simulink model "AssembledTEST1"  (R2016b)
settings: Solver=VariableStepAuto  StartTime=0.0  StopTime=60  RelTol=1e-9
values from neighbouring files (symbols this model uses):
  DOWN_0 = -xtrim(12)    [Comparison_NonLin.m]    (also in InitialiseJ31.m = 1830.0192; Trim.m)
  EAST_0 = xtrim(11)    [Comparison_NonLin.m]    (also in InitialiseJ31.m = 0; Trim.m)
  FLAP = 0    [InitialiseJ31.m]
  INERTIA = [IXX,IXY,IXZ;IXY,IYY,IYZ;IXZ,IYZ,IZZ]    [InitialiseJ31.m]
  NORTH_0 = xtrim(10)    [Comparison_NonLin.m]    (also in InitialiseJ31.m = 0; Trim.m)
  P_0 = xtrim(4)    [Comparison_NonLin.m]    (also in InitialiseJ31.m = 0; Trim.m)
  PHI_0 = xtrim(7)    [Comparison_NonLin.m]    (also in Trim.m)
  PSI_0 = xtrim(9)    [Comparison_NonLin.m]    (also in Trim.m)
  Q_0 = xtrim(5)    [Comparison_NonLin.m]    (also in InitialiseJ31.m = 0; Trim.m)
  R2D = 180/pi    (= 57.2957795131)    [InitialiseJ31.m]
  R_0 = xtrim(6)    [Comparison_NonLin.m]    (also in InitialiseJ31.m = 0; Trim.m)
  THETA_0 = xtrim(8)    [Comparison_NonLin.m]    (also in Trim.m)
  U_0 = xtrim(1)    [Comparison_NonLin.m]    (also in Trim.m)
  V_0 = xtrim(2)    [Comparison_NonLin.m]    (also in Trim.m)
  W_0 = xtrim(3)    [Comparison_NonLin.m]    (also in Trim.m)
undefined symbols (not defined in the file or in its folder): ail_data, Ap, Aw, b, beta0_data, c0, c_i, cdrag_data, CG, clean_wing_data, crt, CT_data, D, D0q_10, D0q_20, D0q_35, DCDi_data, DCM0b, Deh_f_on_data, Deh_on_data, df, Dqhq_data, e0, e_data10, e_data20, e_data35, elaw_0, elaw_1, elaw_2, flaps_lift_data, flaps_moment_data, flaps_tail_data, flaps_wing_data, fmc_data, fmf_data, fmn_data, fus_data, gamma_t, h_data10, h_data20, h_data35, it, iw, Iwn2, J_W, K1_data, k1f_data, k_data, L_r0_10f, L_r0_20f, L_r0_35f, l_t, ld_data, Lt, Lt_dash, Lv_b, Lv_h, Lv_n, mac, mach_ffr ... (+39)
libraries: aerolibasang x3, aerolibatmos2 x1
(part 4 of 5)

== system AssembledTEST1/Subsystem/Powerplants and Slipstream/Subsystem2/Powerplant - port (forces and moments about spinner) (in body axes)/Get_Del_qhq ==
  ab : Inport
  In2 : Inport  Port=2
  eh : Inport  Port=3
  In3 : Inport  Port=4
  eu : Inport  Port=5
  ep : Inport  Port=6
  Abs : Abs
  Add : Sum  Inputs=+-+
  Add2 : Sum  Inputs=--+
  Constant1 : Constant  Value=Xp_dash
  Constant2 : Constant  Value=Lt_dash
  Constant3 : Constant  Value=Z_ht
  Constant4 : Constant  Value=D
  Constant5 : Constant  Value=2
  Constant6 : Constant  Value=Iwn2
  Divide : Product  Inputs=**/
  Embedded MATLAB Function : MATLAB Function  TreatAsAtomicUnit=on
  Embedded MATLAB Function1 : MATLAB Function  TreatAsAtomicUnit=on
  Fcn : Fcn  Expr=tan(u(1))
  Fcn1 : Fcn  Expr=tan(u(1))
  GetDehPower : Lookup2D  RowIndex=eh_off_ords  ColumnIndex=Tc2_ords  Table=Deh_on_data
  GetDehPower_flap : Lookup2D  RowIndex=eh_off_ords  ColumnIndex=Tc2_ords  Table=Deh_f_on_data
  GetDelqhq : Lookup2D  RowIndex=Zh_eff_ords  ColumnIndex=Tc3_ords  Table=Dqhq_data
  Product : Product  RndMeth=Zero
  Product1 : Product  RndMeth=Zero
  Saturation : Saturate  UpperLimit=10  LowerLimit=0  ZeroCross=off
  Saturation1 : Saturate  UpperLimit=2  LowerLimit=0  ZeroCross=off
  deg2rad : Gain  Gain=pi/180
  get_Zh_eff : Sum  Inputs=+-+
  rad2deg : Gain  Gain=180/pi
  Out1 : Outport
  Out2 : Outport  Port=2
  Out3 : Outport  Port=3
  wires:
  In3/1 -> GetDehPower_flap/2, GetDehPower/2, GetDelqhq/2, Embedded MATLAB Function1/3(TC)
  GetDehPower/1 -> Embedded MATLAB Function/2(Deh_power)
  GetDehPower_flap/1 -> Embedded MATLAB Function/3(Deh_power_flap)
  In2/1 -> Embedded MATLAB Function/1(Flap)
  rad2deg/1 -> GetDehPower/1, GetDehPower_flap/1
  eh/1 -> rad2deg/1, Add2/2
  eu/1 -> Add/1, Embedded MATLAB Function1/2(eu)
  ep/1 -> Add/2, Embedded MATLAB Function1/1(ep)
  ab/1 -> Add/3
  deg2rad/1 -> Add2/1, Out2/1
  Add/1 -> Fcn/1, Add2/3
  Constant1/1 -> Product/1
  Fcn/1 -> Product/2
  Add2/1 -> Fcn1/1
  Constant2/1 -> Product1/1
  Fcn1/1 -> Product1/2
  Product1/1 -> get_Zh_eff/1
  Constant3/1 -> get_Zh_eff/2
  Product/1 -> get_Zh_eff/3
  get_Zh_eff/1 -> Abs/1
  Embedded MATLAB Function/1(Del_eh_power) -> Saturation/1
  Saturation/1 -> deg2rad/1
  Abs/1 -> Divide/1
  Constant5/1 -> Divide/2
  Constant4/1 -> Divide/3
  Divide/1 -> GetDelqhq/1
  GetDelqhq/1 -> Saturation1/1
  Saturation1/1 -> Out1/1
  Constant6/1 -> Embedded MATLAB Function1/4(Iwn2)
  Embedded MATLAB Function1/1(DelMp_q) -> Out3/1

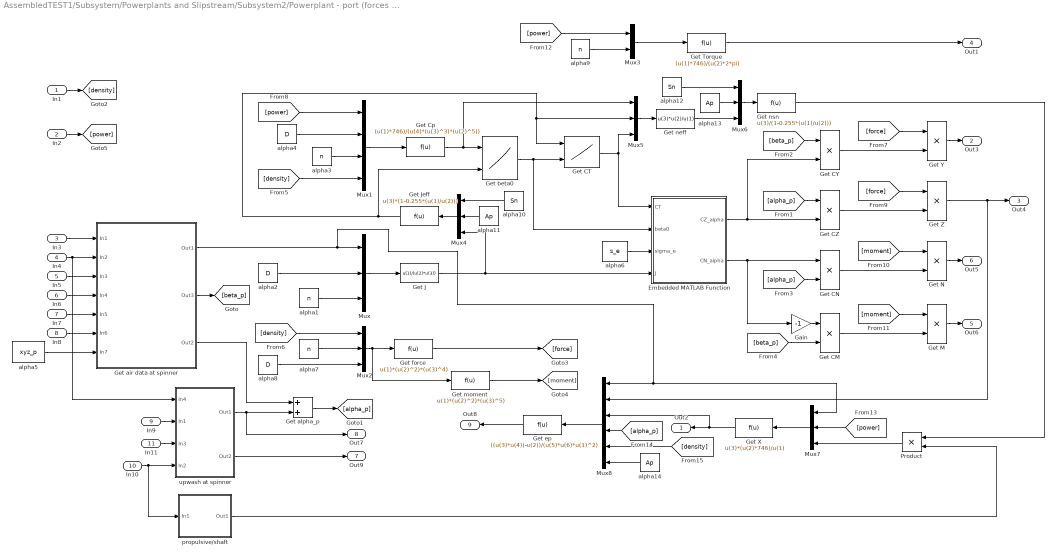
== system AssembledTEST1/Subsystem/Powerplants and Slipstream/Subsystem2/Powerplant - port (forces and moments about spinner) (in body axes)/Propeller - left (forces and moments about spinner) (in body axes) ==
  In1 : Inport
  In2 : Inport  Port=2
  In3 : Inport  Port=3
  In4 : Inport  Port=4
  In5 : Inport  Port=5
  In6 : Inport  Port=6
  In7 : Inport  Port=7
  In8 : Inport  Port=8
  In9 : Inport  Port=9
  In10 : Inport  Port=10
  In11 : Inport  Port=11
  Embedded MATLAB Function : MATLAB Function  TreatAsAtomicUnit=on
  Gain : Gain  Gain=-1
  Get CM : Product  RndMeth=Zero
  Get CN : Product  RndMeth=Zero
  Get CT : Lookup2D  RowIndex=J_ords  ColumnIndex=beta0_ords  Table=CT_data
  Get CY : Product  RndMeth=Zero
  Get CZ : Product  RndMeth=Zero
  Get Cp : Fcn  Expr=(u(1)*746)/(u(4)*(u(3)^3)*(u(2)^5))
  Get J : Fcn  Expr=u(1)/(u(2)*u(3))
  Get Jeff : Fcn  Expr=u(3)*(1-0.255*(u(1)/u(2)))
  Get M : Product  RndMeth=Zero
  Get N : Product  RndMeth=Zero
  Get Torque : Fcn  Expr=(u(1)*746)/(u(2)*2*pi)
  Get X : Fcn  Expr=u(3)*(u(2)*746)/u(1)
  Get Y : Product  RndMeth=Zero
  Get Z : Product  RndMeth=Zero
  Get air data at spinner : Subsystem
      mask Display:
      | port_label('input',1,'V_b [m/s]','texmode','on')
      | port_label('output',1,'V_p [m/s]','texmode','on')
      | port_label('input',2,'\alpha_b [rad/s]','texmode','on')
      | port_label('input',3,'\beta_b [rad/s]','texmode','on')
      | port_label('output',3,'\alpha_s [rad]','texmode','on')
      | port_label('output',2,'\beta_p [rad]','texmode','on')
      | port_label('input',4,'p [rad/s]')
      | port_label('input',5,'q [rad/s]')
      | port_label('input',6,'r [rad/s]')
      | port_label('input',7,'spinner location [m]','texmode','on')
  Get alpha_p : Sum
  Get beta0 : Lookup2D  RowIndex=CP_ords  ColumnIndex=J_ords  Table=beta0_data
  Get ep : Fcn  Expr=((u(3)*u(4))-u(2))/(u(5)*u(6)*u(1)^2)
  "Get force " : Fcn  Expr=u(1)*(u(2)^2)*(u(3)^4)
  Get moment : Fcn  Expr=u(1)*(u(2)^2)*(u(3)^5)
  Get neff : Fcn  Expr=u(3)*u(2)/u(1)
  Get nsn : Fcn  Expr=u(3)/(1-0.255*(u(1)/u(2)))
  Mux{,2,4..7} (6 alike) : Mux  Inputs=3
  Mux1 : Mux
  Mux3 : Mux  Inputs=2
  Mux8 : Mux  Inputs=6
  Product : Product  RndMeth=Zero
  alpha{1,3,7,9} (4 alike) : Constant  Value=n
  alpha10 : Constant  Value=Sn
  alpha11 : Constant  Value=Ap
  alpha12 : Constant  Value=Sn
  alpha13 : Constant  Value=Ap
  alpha14 : Constant  Value=Ap
  alpha2 : Constant  Value=D
  alpha4 : Constant  Value=D
  alpha5 : Constant  Value=xyz_p
  alpha6 : Constant  Value=s_e
  alpha8 : Constant  Value=D
  propulsive/shaft : Subsystem
      mask Display:
      | port_label('input',1,'Mach')
      | port_label('output',1,'\eta_{Pn}/\eta_{Sn}','texmode','on')
  upwash at spinner : Subsystem
      mask Display:
      | port_label('input',2,'Flap')
      | port_label('input',4,'Mach')
      | port_label('input',3,'C_L','texmode','on')
      | port_label('input',1,'\alpha_b','texmode','on')
      | port_label('output',1,'\epsilon_u','texmode','on')
      | port_label('output',2,'\delta\epsilon_u/\deltaC_L','texmode','on')
  Out2 : Outport
  Out3 : Outport  Port=2
  Out4 : Outport  Port=3
  Out1 : Outport  Port=4
  Out6 : Outport  Port=5
  Out5 : Outport  Port=6
  Out9 : Outport  Port=7
  Out7 : Outport  Port=8
  Out8 : Outport  Port=9
  wires:
  alpha2/1 -> Mux/2
  alpha1/1 -> Mux/3
  Mux/1 -> Get J/1
  alpha4/1 -> Mux1/2
  alpha3/1 -> Mux1/3
  Mux1/1 -> Get Cp/1
  Get beta0/1 -> Get CT/2, Embedded MATLAB Function/2(beta0)
  Get Cp/1 -> Get beta0/1, Mux5/1
  Get J/1 -> Embedded MATLAB Function/4(J), Mux4/3
  Get CT/1 -> Embedded MATLAB Function/1(CT), Mux5/3
  alpha5/1 -> Get air data at spinner/7(In7)
  Get air data at spinner/3(Out2) -> Get alpha_p/1
  Get air data at spinner/2(Out3) -> [beta_p]
  In5/1 -> Get air data at spinner/3(In3)
  Get air data at spinner/1(Out1) -> Mux/1, Mux7/1, Mux8/1
  alpha6/1 -> Embedded MATLAB Function/3(sigma_e)
  Embedded MATLAB Function/1(CZ_alpha) -> Get CZ/2, Get CY/2
  upwash at spinner/1(Out1) -> Get alpha_p/2, Out7/1
  Get alpha_p/1 -> [alpha_p]
  [alpha_p] -> Get CZ/1
  [beta_p] -> Get CY/1
  Embedded MATLAB Function/2(CN_alpha) -> Get CN/1, Gain/1
  [alpha_p] -> Get CN/2
  Gain/1 -> Get CM/1
  [beta_p] -> Get CM/2
  [density] -> Mux1/4
  [density] -> Mux2/1
  alpha7/1 -> Mux2/2
  alpha8/1 -> Mux2/3
  Mux2/1 -> "Get force "/1, Get moment/1
  "Get force "/1 -> [force]
  Get moment/1 -> [moment]
  [force] -> Get Y/1
  Get CY/1 -> Get Y/2
  [force] -> Get Z/1
  Get CZ/1 -> Get Z/2
  [moment] -> Get N/1
  Get CN/1 -> Get N/2
  [moment] -> Get M/1
  Get CM/1 -> Get M/2
  Get Torque/1 -> Out1/1
  In1/1 -> [density]
  Get Y/1 -> Out3/1
  Get Z/1 -> Out4/1, Mux8/2
  In3/1 -> Get air data at spinner/1(In1)
  In4/1 -> Get air data at spinner/2(In2), upwash at spinner/1(In4)
  Get N/1 -> Out5/1
  In6/1 -> Get air data at spinner/4(In4)
  In7/1 -> Get air data at spinner/5(In5)
  In8/1 -> Get air data at spinner/6(In6)
  Get M/1 -> Out6/1
  In9/1 -> upwash at spinner/2(In1)
  In10/1 -> upwash at spinner/4(In2), propulsive/shaft/1(In1)
  In11/1 -> upwash at spinner/3(In3)
  Mux3/1 -> Get Torque/1
  alpha9/1 -> Mux3/2
  alpha10/1 -> Mux4/1
  Mux4/1 -> Get Jeff/1
  alpha11/1 -> Mux4/2
  Get Jeff/1 -> Get beta0/2, Get CT/1, Mux5/2
  Mux5/1 -> Get neff/1
  alpha12/1 -> Mux6/1
  Mux6/1 -> Get nsn/1
  alpha13/1 -> Mux6/2
  Get neff/1 -> Mux6/3
  Get nsn/1 -> Product/1
  propulsive/shaft/1(Out1) -> Product/2
  In2/1 -> [power]
  [power] -> Mux1/1
  [power] -> Mux3/1
  Get X/1 -> Out2/1, Mux8/3
  Mux7/1 -> Get X/1
  [power] -> Mux7/2
  Product/1 -> Mux7/3
  Mux8/1 -> Get ep/1
  Get ep/1 -> Out8/1
  [alpha_p] -> Mux8/4
  [density] -> Mux8/5
  upwash at spinner/2(Out2) -> Out9/1
  alpha14/1 -> Mux8/6

== system AssembledTEST1/Subsystem/Powerplants and Slipstream/Subsystem2/Powerplant - port (forces and moments about spinner) (in body axes)/get_D0//q_flap ==
  flap : Inport
  Constant1 : Constant  Value=0
  Constant2 : Constant  Value=D0q_10
  Constant3 : Constant  Value=D0q_20
  Constant4 : Constant  Value=D0q_35
  Multiport Switch : MultiPortSwitch  Inputs=4
  D0q_flap : Outport
  wires:
  Constant1/1 -> Multiport Switch/2
  Constant2/1 -> Multiport Switch/3
  Constant3/1 -> Multiport Switch/4
  Constant4/1 -> Multiport Switch/5
  flap/1 -> Multiport Switch/1
  Multiport Switch/1 -> D0q_flap/1

== system AssembledTEST1/Subsystem/Powerplants and Slipstream/Subsystem2/Powerplant - port (forces and moments about spinner) (in body axes)/get_a1 ==
  flap : Inport
  Mach : Inport  Port=2
  Multiport Switch : MultiPortSwitch  Inputs=4
  a1_clean : Lookup  InputValues=clean_wing_data(:,1)  Table=clean_wing_data(:,2)
  a1_flaps10 : Lookup  InputValues=flaps_wing_data(:,1)  Table=flaps_wing_data(:,3)
  a1_flaps20 : Lookup  InputValues=flaps_wing_data(:,1)  Table=flaps_wing_data(:,6)
  a1_flaps35 : Lookup  InputValues=flaps_wing_data(:,1)  Table=flaps_wing_data(:,9)
  a1 : Outport
  wires:
  Mach/1 -> a1_flaps35/1, a1_flaps20/1, a1_flaps10/1, a1_clean/1
  a1_clean/1 -> Multiport Switch/2
  a1_flaps10/1 -> Multiport Switch/3
  a1_flaps20/1 -> Multiport Switch/4
  a1_flaps35/1 -> Multiport Switch/5
  flap/1 -> Multiport Switch/1
  Multiport Switch/1 -> a1/1

== system AssembledTEST1/Subsystem/Powerplants and Slipstream/Subsystem2/Powerplant - starboard (forces and moments about spinner) (in body axes)/Engine ==
  In2 : Inport
  In1 : Inport  Port=2
  In3 : Inport  Port=3
  In4 : Inport  Port=4
  % throttle to FFR : Gain  Gain=2.5
  Altitude effect on FFR : Fcn  Expr=u(3)*u(2)*sqrt(u(1))
  Altitude effect on power : Fcn  Expr=u(3)*u(2)*sqrt(u(1))
  Constant10 : Constant  Value=mach_pow
  Constant4 : Constant  Value=mach_ffr
  Constant5 : Constant  Value=288.15
  Constant6 : Constant  Value=101325
  Constant7 : Constant  Value=elaw_2
  Constant8 : Constant  Value=elaw_1
  Constant9 : Constant  Value=elaw_0
  Divide : Product  Inputs=*/
  Divide1 : Product  Inputs=*/
  FFR law : Fcn  Expr=(u(2)*u(1)^2)+(u(3)*u(1))+u(4)
  Mach effect on FFR : Fcn  Expr=u(3)*(1+u(2)*u(1)^2)
  Mach effect on power : Fcn  Expr=u(3)*(1+u(2)*u(1)^2)
  Mux : Mux
  Mux{1..4} (4 alike) : Mux  Inputs=3
  Out1 : Outport
  Out2 : Outport  Port=2
  wires:
  Constant5/1 -> Divide/2
  Constant6/1 -> Divide1/2
  % throttle to FFR/1 -> Mux/1, Mux1/3
  Constant7/1 -> Mux/2
  Constant8/1 -> Mux/3
  Constant9/1 -> Mux/4
  Mux/1 -> FFR law/1
  Mux1/1 -> Mach effect on FFR/1
  Constant4/1 -> Mux1/2
  Mux2/1 -> Mach effect on power/1
  Constant10/1 -> Mux2/2
  FFR law/1 -> Mux2/3
  Divide/1 -> [theta]
  Divide1/1 -> [delta]
  [Mach] -> Mux1/1
  [Mach] -> Mux2/1
  Mux3/1 -> Altitude effect on FFR/1
  [theta] -> Mux3/1
  [delta] -> Mux3/2
  Mach effect on FFR/1 -> Mux3/3
  Mux4/1 -> Altitude effect on power/1
  [theta] -> Mux4/1
  [delta] -> Mux4/2
  Mach effect on power/1 -> Mux4/3
  In1/1 -> Divide1/1
  In2/1 -> [Mach]
  In3/1 -> Divide/1
  Altitude effect on FFR/1 -> Out1/1
  Altitude effect on power/1 -> Out2/1
  In4/1 -> % throttle to FFR/1

== system AssembledTEST1/Subsystem/Powerplants and Slipstream/Subsystem2/Powerplant - starboard (forces and moments about spinner) (in body axes)/Get_Del_qhq ==
  ab : Inport
  In2 : Inport  Port=2
  eh : Inport  Port=3
  In3 : Inport  Port=4
  eu : Inport  Port=5
  ep : Inport  Port=6
  Abs : Abs
  Add : Sum  Inputs=+-+
  Add2 : Sum  Inputs=--+
  Constant1 : Constant  Value=Xp_dash
  Constant2 : Constant  Value=Lt_dash
  Constant3 : Constant  Value=Z_ht
  Constant4 : Constant  Value=D
  Constant5 : Constant  Value=2
  Constant6 : Constant  Value=Iwn2
  Divide : Product  Inputs=**/
  Embedded MATLAB Function : MATLAB Function  TreatAsAtomicUnit=on
  Embedded MATLAB Function1 : MATLAB Function  TreatAsAtomicUnit=on
  Fcn : Fcn  Expr=tan(u(1))
  Fcn1 : Fcn  Expr=tan(u(1))
  GetDehPower : Lookup2D  RowIndex=eh_off_ords  ColumnIndex=Tc2_ords  Table=Deh_on_data
  GetDehPower_flap : Lookup2D  RowIndex=eh_off_ords  ColumnIndex=Tc2_ords  Table=Deh_f_on_data
  GetDelqhq : Lookup2D  RowIndex=Zh_eff_ords  ColumnIndex=Tc3_ords  Table=Dqhq_data
  Product : Product  RndMeth=Zero
  Product1 : Product  RndMeth=Zero
  Saturation : Saturate  UpperLimit=10  LowerLimit=0  ZeroCross=off
  Saturation1 : Saturate  UpperLimit=2  LowerLimit=0  ZeroCross=off
  deg2rad : Gain  Gain=pi/180
  get_Zh_eff : Sum  Inputs=+-+
  rad2deg : Gain  Gain=180/pi
  Out1 : Outport
  Out2 : Outport  Port=2
  Out3 : Outport  Port=3
  wires:
  In3/1 -> GetDehPower_flap/2, GetDehPower/2, GetDelqhq/2, Embedded MATLAB Function1/3(TC)
  GetDehPower/1 -> Embedded MATLAB Function/2(Deh_power)
  GetDehPower_flap/1 -> Embedded MATLAB Function/3(Deh_power_flap)
  In2/1 -> Embedded MATLAB Function/1(Flap)
  rad2deg/1 -> GetDehPower/1, GetDehPower_flap/1
  eh/1 -> rad2deg/1, Add2/2
  eu/1 -> Add/1, Embedded MATLAB Function1/2(eu)
  ep/1 -> Add/2, Embedded MATLAB Function1/1(ep)
  ab/1 -> Add/3
  deg2rad/1 -> Add2/1, Out2/1
  Add/1 -> Fcn/1, Add2/3
  Constant1/1 -> Product/1
  Fcn/1 -> Product/2
  Add2/1 -> Fcn1/1
  Constant2/1 -> Product1/1
  Fcn1/1 -> Product1/2
  Product1/1 -> get_Zh_eff/1
  Constant3/1 -> get_Zh_eff/2
  Product/1 -> get_Zh_eff/3
  get_Zh_eff/1 -> Abs/1
  Embedded MATLAB Function/1(Del_eh_power) -> Saturation/1
  Saturation/1 -> deg2rad/1
  Abs/1 -> Divide/1
  Constant5/1 -> Divide/2
  Constant4/1 -> Divide/3
  Divide/1 -> GetDelqhq/1
  GetDelqhq/1 -> Saturation1/1
  Saturation1/1 -> Out1/1
  Constant6/1 -> Embedded MATLAB Function1/4(Iwn2)
  Embedded MATLAB Function1/1(DelMp_q) -> Out3/1

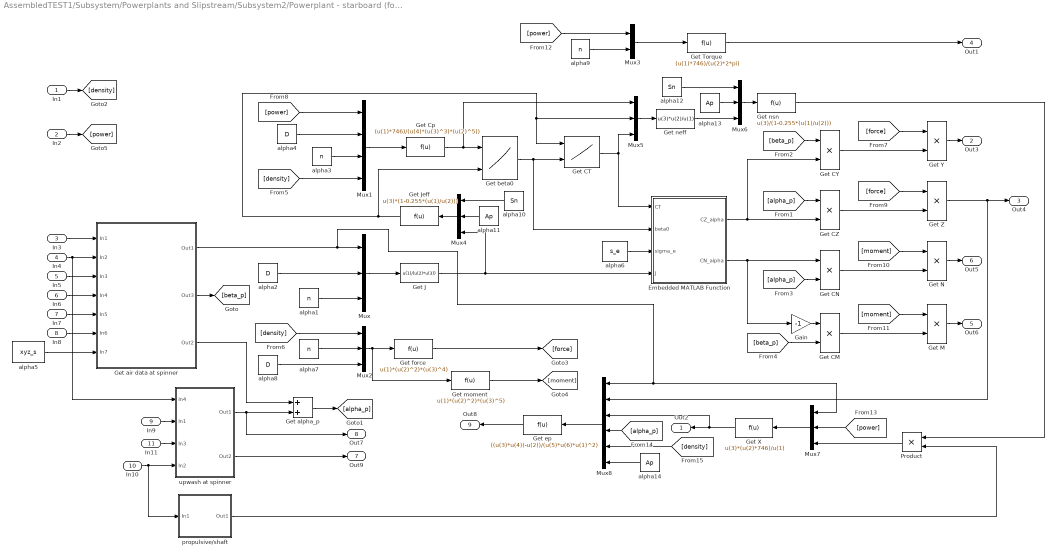
== system AssembledTEST1/Subsystem/Powerplants and Slipstream/Subsystem2/Powerplant - starboard (forces and moments about spinner) (in body axes)/Propeller - right (forces and moments about spinner) (in body axes) ==
  In1 : Inport
  In2 : Inport  Port=2
  In3 : Inport  Port=3
  In4 : Inport  Port=4
  In5 : Inport  Port=5
  In6 : Inport  Port=6
  In7 : Inport  Port=7
  In8 : Inport  Port=8
  In9 : Inport  Port=9
  In10 : Inport  Port=10
  In11 : Inport  Port=11
  Embedded MATLAB Function : MATLAB Function  TreatAsAtomicUnit=on
  Gain : Gain  Gain=-1
  Get CM : Product  RndMeth=Zero
  Get CN : Product  RndMeth=Zero
  Get CT : Lookup2D  RowIndex=J_ords  ColumnIndex=beta0_ords  Table=CT_data
  Get CY : Product  RndMeth=Zero
  Get CZ : Product  RndMeth=Zero
  Get Cp : Fcn  Expr=(u(1)*746)/(u(4)*(u(3)^3)*(u(2)^5))
  Get J : Fcn  Expr=u(1)/(u(2)*u(3))
  Get Jeff : Fcn  Expr=u(3)*(1-0.255*(u(1)/u(2)))
  Get M : Product  RndMeth=Zero
  Get N : Product  RndMeth=Zero
  Get Torque : Fcn  Expr=(u(1)*746)/(u(2)*2*pi)
  Get X : Fcn  Expr=u(3)*(u(2)*746)/u(1)
  Get Y : Product  RndMeth=Zero
  Get Z : Product  RndMeth=Zero
  Get air data at spinner : Subsystem
      mask Display:
      | port_label('input',1,'V_b [m/s]','texmode','on')
      | port_label('output',1,'V_p [m/s]','texmode','on')
      | port_label('input',2,'\alpha_b [rad/s]','texmode','on')
      | port_label('input',3,'\beta_b [rad/s]','texmode','on')
      | port_label('output',3,'\alpha_s [rad]','texmode','on')
      | port_label('output',2,'\beta_p [rad]','texmode','on')
      | port_label('input',4,'p [rad/s]')
      | port_label('input',5,'q [rad/s]')
      | port_label('input',6,'r [rad/s]')
      | port_label('input',7,'spinner location [m]','texmode','on')
  Get alpha_p : Sum
  Get beta0 : Lookup2D  RowIndex=CP_ords  ColumnIndex=J_ords  Table=beta0_data
  Get ep : Fcn  Expr=((u(3)*u(4))-u(2))/(u(5)*u(6)*u(1)^2)
  "Get force " : Fcn  Expr=u(1)*(u(2)^2)*(u(3)^4)
  Get moment : Fcn  Expr=u(1)*(u(2)^2)*(u(3)^5)
  Get neff : Fcn  Expr=u(3)*u(2)/u(1)
  Get nsn : Fcn  Expr=u(3)/(1-0.255*(u(1)/u(2)))
  Mux{,2,4..7} (6 alike) : Mux  Inputs=3
  Mux1 : Mux
  Mux3 : Mux  Inputs=2
  Mux8 : Mux  Inputs=6
  Product : Product  RndMeth=Zero
  alpha{1,3,7,9} (4 alike) : Constant  Value=n
  alpha10 : Constant  Value=Sn
  alpha11 : Constant  Value=Ap
  alpha12 : Constant  Value=Sn
  alpha13 : Constant  Value=Ap
  alpha14 : Constant  Value=Ap
  alpha2 : Constant  Value=D
  alpha4 : Constant  Value=D
  alpha5 : Constant  Value=xyz_s
  alpha6 : Constant  Value=s_e
  alpha8 : Constant  Value=D
  propulsive/shaft : Subsystem
      mask Display:
      | port_label('input',1,'Mach')
      | port_label('output',1,'\eta_{Pn}/\eta_{Sn}','texmode','on')
  upwash at spinner : Subsystem
      mask Display:
      | port_label('input',2,'Flap')
      | port_label('input',4,'Mach')
      | port_label('input',3,'C_L','texmode','on')
      | port_label('input',1,'\alpha_b','texmode','on')
      | port_label('output',1,'\epsilon_u','texmode','on')
      | port_label('output',2,'\delta\epsilon_u/\deltaC_L','texmode','on')
  Out2 : Outport
  Out3 : Outport  Port=2
  Out4 : Outport  Port=3
  Out1 : Outport  Port=4
  Out6 : Outport  Port=5
  Out5 : Outport  Port=6
  Out9 : Outport  Port=7
  Out7 : Outport  Port=8
  Out8 : Outport  Port=9
  wires:
  alpha2/1 -> Mux/2
  alpha1/1 -> Mux/3
  Mux/1 -> Get J/1
  alpha4/1 -> Mux1/2
  alpha3/1 -> Mux1/3
  Mux1/1 -> Get Cp/1
  Get beta0/1 -> Get CT/2, Embedded MATLAB Function/2(beta0)
  Get Cp/1 -> Get beta0/1, Mux5/1
  Get J/1 -> Embedded MATLAB Function/4(J), Mux4/3
  Get CT/1 -> Embedded MATLAB Function/1(CT), Mux5/3
  alpha5/1 -> Get air data at spinner/7(In7)
  Get air data at spinner/3(Out2) -> Get alpha_p/1
  Get air data at spinner/2(Out3) -> [beta_p]
  In5/1 -> Get air data at spinner/3(In3)
  Get air data at spinner/1(Out1) -> Mux/1, Mux7/1, Mux8/1
  alpha6/1 -> Embedded MATLAB Function/3(sigma_e)
  Embedded MATLAB Function/1(CZ_alpha) -> Get CZ/2, Get CY/2
  upwash at spinner/1(Out1) -> Get alpha_p/2, Out7/1
  Get alpha_p/1 -> [alpha_p]
  [alpha_p] -> Get CZ/1
  [beta_p] -> Get CY/1
  Embedded MATLAB Function/2(CN_alpha) -> Get CN/1, Gain/1
  [alpha_p] -> Get CN/2
  Gain/1 -> Get CM/1
  [beta_p] -> Get CM/2
  [density] -> Mux1/4
  [density] -> Mux2/1
  alpha7/1 -> Mux2/2
  alpha8/1 -> Mux2/3
  Mux2/1 -> "Get force "/1, Get moment/1
  "Get force "/1 -> [force]
  Get moment/1 -> [moment]
  [force] -> Get Y/1
  Get CY/1 -> Get Y/2
  [force] -> Get Z/1
  Get CZ/1 -> Get Z/2
  [moment] -> Get N/1
  Get CN/1 -> Get N/2
  [moment] -> Get M/1
  Get CM/1 -> Get M/2
  Get Torque/1 -> Out1/1
  In1/1 -> [density]
  Get Y/1 -> Out3/1
  Get Z/1 -> Out4/1, Mux8/2
  In3/1 -> Get air data at spinner/1(In1)
  In4/1 -> Get air data at spinner/2(In2), upwash at spinner/1(In4)
  Get N/1 -> Out5/1
  In6/1 -> Get air data at spinner/4(In4)
  In7/1 -> Get air data at spinner/5(In5)
  In8/1 -> Get air data at spinner/6(In6)
  Get M/1 -> Out6/1
  In9/1 -> upwash at spinner/2(In1)
  In10/1 -> upwash at spinner/4(In2), propulsive/shaft/1(In1)
  In11/1 -> upwash at spinner/3(In3)
  Mux3/1 -> Get Torque/1
  alpha9/1 -> Mux3/2
  alpha10/1 -> Mux4/1
  Mux4/1 -> Get Jeff/1
  alpha11/1 -> Mux4/2
  Get Jeff/1 -> Get beta0/2, Get CT/1, Mux5/2
  Mux5/1 -> Get neff/1
  alpha12/1 -> Mux6/1
  Mux6/1 -> Get nsn/1
  alpha13/1 -> Mux6/2
  Get neff/1 -> Mux6/3
  Get nsn/1 -> Product/1
  propulsive/shaft/1(Out1) -> Product/2
  In2/1 -> [power]
  [power] -> Mux1/1
  [power] -> Mux3/1
  Get X/1 -> Out2/1, Mux8/3
  Mux7/1 -> Get X/1
  [power] -> Mux7/2
  Product/1 -> Mux7/3
  Mux8/1 -> Get ep/1
  Get ep/1 -> Out8/1
  [alpha_p] -> Mux8/4
  [density] -> Mux8/5
  upwash at spinner/2(Out2) -> Out9/1
  alpha14/1 -> Mux8/6

== system AssembledTEST1/Subsystem/Powerplants and Slipstream/Subsystem2/Powerplant - starboard (forces and moments about spinner) (in body axes)/get_D0//q_flap ==
  flap : Inport
  Constant1 : Constant  Value=0
  Constant2 : Constant  Value=D0q_10
  Constant3 : Constant  Value=D0q_20
  Constant4 : Constant  Value=D0q_35
  Multiport Switch : MultiPortSwitch  Inputs=4
  D0q_flap : Outport
  wires:
  Constant1/1 -> Multiport Switch/2
  Constant2/1 -> Multiport Switch/3
  Constant3/1 -> Multiport Switch/4
  Constant4/1 -> Multiport Switch/5
  flap/1 -> Multiport Switch/1
  Multiport Switch/1 -> D0q_flap/1

== system AssembledTEST1/Subsystem/Powerplants and Slipstream/Subsystem2/Powerplant - starboard (forces and moments about spinner) (in body axes)/get_a1 ==
  flap : Inport
  Mach : Inport  Port=2
  Multiport Switch : MultiPortSwitch  Inputs=4
  a1_clean : Lookup  InputValues=clean_wing_data(:,1)  Table=clean_wing_data(:,2)
  a1_flaps10 : Lookup  InputValues=flaps_wing_data(:,1)  Table=flaps_wing_data(:,3)
  a1_flaps20 : Lookup  InputValues=flaps_wing_data(:,1)  Table=flaps_wing_data(:,6)
  a1_flaps35 : Lookup  InputValues=flaps_wing_data(:,1)  Table=flaps_wing_data(:,9)
  a1 : Outport
  wires:
  Mach/1 -> a1_flaps35/1, a1_flaps20/1, a1_flaps10/1, a1_clean/1
  a1_clean/1 -> Multiport Switch/2
  a1_flaps10/1 -> Multiport Switch/3
  a1_flaps20/1 -> Multiport Switch/4
  a1_flaps35/1 -> Multiport Switch/5
  flap/1 -> Multiport Switch/1
  Multiport Switch/1 -> a1/1

== system AssembledTEST1/Subsystem/Powerplants and Slipstream/Subsystem2/Powerplant - port (forces and moments about spinner) (in body axes)/Propeller - left (forces and moments about spinner) (in body axes)/Get air data at spinner ==
  In1 : Inport
  In2 : Inport  Port=2
  In3 : Inport  Port=3
  In4 : Inport  Port=4
  In5 : Inport  Port=5
  In6 : Inport  Port=6
  In7 : Inport  Port=7
  Add : Sum
  Display : Display
  Gain : Gain  Gain=-1
  Gain1 : Gain  Gain=-1
  Gain2 : Gain  Gain=-1
  Ground : Ground
  Ground1 : Ground
  Ground2 : Ground
  Matrix Concatenation{,1..3} (4 alike) : Concatenate  NumInputs=3  Mode=Multidimensional array
  Matrix Concatenation4 : Concatenate  NumInputs=3  Mode=Multidimensional array  ConcatenateDimension=2
  Mux2 : Mux  Inputs=2
  Product : Product  Inputs=**  Multiplication=Matrix(*)  RndMeth=Zero
  Trigonometric Function : Trigonometry
  Trigonometric Function1 : Trigonometry  Operator=cos
  Trigonometric Function2 : Trigonometry
  Trigonometric Function3 : Trigonometry  Operator=cos
  V_p : Fcn  Expr=sqrt(u(1)^2+u(2)^2+u(3)^2)
  alpha_p : Fcn  Expr=atan(u(4)/u(2))
  beta_p : Fcn  Expr=asin(u(3)/u(1))
  ub : Product  Inputs=3  RndMeth=Zero
  vb : Product  RndMeth=Zero
  wb : Product  Inputs=3  RndMeth=Zero
  Out1 : Outport
  Out3 : Outport  Port=2
  Out2 : Outport  Port=3
  wires:
  In2/1 -> Trigonometric Function1/1, Trigonometric Function/1
  In3/1 -> Trigonometric Function3/1, Trigonometric Function2/1
  Trigonometric Function1/1 -> ub/1
  Trigonometric Function3/1 -> ub/2, wb/2
  [V] -> ub/3
  Trigonometric Function/1 -> wb/1
  [V] -> wb/3
  Trigonometric Function2/1 -> vb/1
  [V] -> vb/2
  ub/1 -> Matrix Concatenation/1
  vb/1 -> Matrix Concatenation/2
  wb/1 -> Matrix Concatenation/3
  Ground/1 -> Matrix Concatenation1/1
  Gain/1 -> Matrix Concatenation1/3
  [r] -> Matrix Concatenation1/2
  [q] -> Gain/1
  [r] -> Gain1/1
  Gain1/1 -> Matrix Concatenation2/1
  Ground1/1 -> Matrix Concatenation2/2
  [p] -> Matrix Concatenation2/3
  [p] -> Gain2/1
  [q] -> Matrix Concatenation3/1
  Gain2/1 -> Matrix Concatenation3/2
  Ground2/1 -> Matrix Concatenation3/3
  Matrix Concatenation1/1 -> Matrix Concatenation4/1
  Matrix Concatenation2/1 -> Matrix Concatenation4/2
  Matrix Concatenation3/1 -> Matrix Concatenation4/3
  Matrix Concatenation4/1 -> Product/1
  Product/1 -> Add/2
  Matrix Concatenation/1 -> Add/1
  Add/1 -> V_p/1, Mux2/2
  V_p/1 -> Mux2/1, Out1/1
  Mux2/1 -> alpha_p/1, beta_p/1, Display/1
  In1/1 -> [V]
  In4/1 -> [p]
  In5/1 -> [q]
  alpha_p/1 -> Out2/1
  In6/1 -> [r]
  beta_p/1 -> Out3/1
  In7/1 -> Product/2

== system AssembledTEST1/Subsystem/Powerplants and Slipstream/Subsystem2/Powerplant - port (forces and moments about spinner) (in body axes)/Propeller - left (forces and moments about spinner) (in body axes)/propulsive//shaft ==
  In1 : Inport
  D0/q nacelles : Lookup  InputValues=pdrag_data(:,1)  Table=pdrag_data(:,6)
  Divide : Product  Inputs=*//
  Mux : Mux  Inputs=3
  alpha1 : Constant  Value=Ap
  alpha14 : Constant  Value=Sn
  alpha15 : Constant  Value=2
  propulsive/shaft : Fcn  Expr=1-(0.5*(u(3)/u(2))*((2.4*u(1))+0.51))
  Out1 : Outport
  wires:
  D0/q nacelles/1 -> Divide/1
  In1/1 -> D0/q nacelles/1
  alpha15/1 -> Divide/2
  alpha14/1 -> Divide/3, Mux/3
  Divide/1 -> Mux/1
  Mux/1 -> propulsive/shaft/1
  propulsive/shaft/1 -> Out1/1
  alpha1/1 -> Mux/2

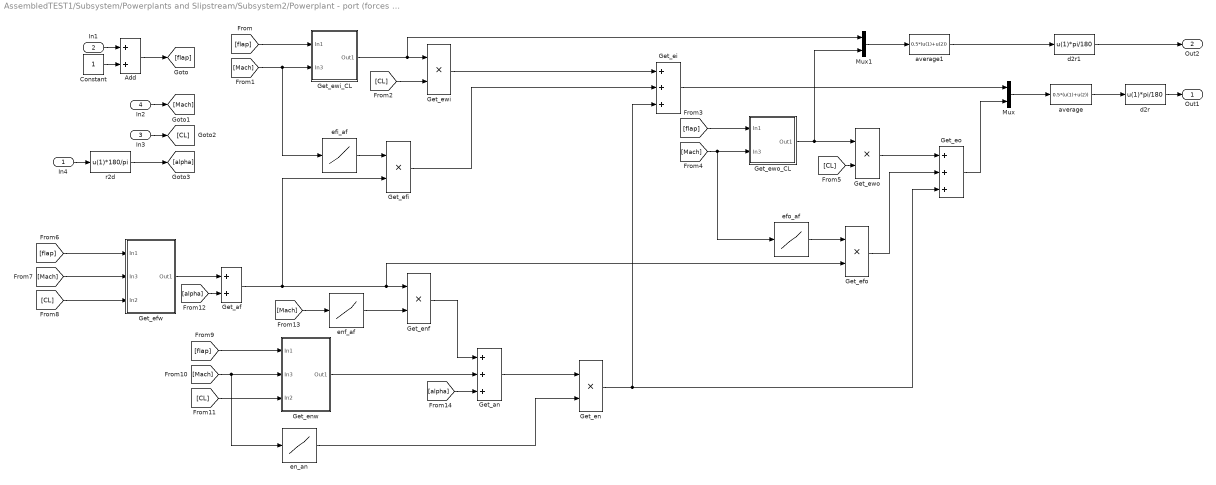
== system AssembledTEST1/Subsystem/Powerplants and Slipstream/Subsystem2/Powerplant - port (forces and moments about spinner) (in body axes)/Propeller - left (forces and moments about spinner) (in body axes)/upwash at spinner ==
  In4 : Inport
  In1 : Inport  Port=2
  In3 : Inport  Port=3
  In2 : Inport  Port=4
  Add : Sum
  Constant : Constant
  Get_af : Sum
  Get_an : Sum  Inputs=+++
  Get_efi : Product  RndMeth=Zero
  Get_efo : Product  RndMeth=Zero
  Get_efw : Subsystem
      mask Display:
      | port_label('output',1,'\epsilon^f_{w}','texmode','on')
      | port_label('input',1,'flap')
      | port_label('input',2,'Mach')
      | port_label('input',3,'C_L','texmode','on')
  Get_ei : Sum  Inputs=+++
  Get_en : Product  RndMeth=Zero
  Get_enf : Product  RndMeth=Zero
  Get_enw : Subsystem
      mask Display:
      | port_label('output',1,'\epsilon^n_{w}','texmode','on')
      | port_label('input',1,'flap')
      | port_label('input',2,'Mach')
      | port_label('input',3,'C_L','texmode','on')
  Get_eo : Sum  Inputs=+++
  Get_ewi : Product  RndMeth=Zero
  Get_ewi_CL : Subsystem
      mask Display:
      | port_label('output',1,'\epsilon_{wi}/C_L','texmode','on')
      | port_label('input',1,'flap')
      | port_label('input',2,'Mach')
  Get_ewo : Product  RndMeth=Zero
  Get_ewo_CL : Subsystem
      mask Display:
      | port_label('output',1,'\epsilon_{wo}/C_L','texmode','on')
      | port_label('input',1,'flap')
      | port_label('input',2,'Mach')
  Mux : Mux  Inputs=2
  Mux1 : Mux  Inputs=2
  average : Fcn  Expr=0.5*(u(1)+u(2))
  average1 : Fcn  Expr=0.5*(u(1)+u(2))
  d2r : Fcn  Expr=u(1)*pi/180
  d2r1 : Fcn  Expr=u(1)*pi/180
  efi_af : Lookup  InputValues=upwash_clean(:,1)  Table=upwash_clean(:,6)
  efo_af : Lookup  InputValues=upwash_clean(:,1)  Table=upwash_clean(:,7)
  en_an : Lookup  InputValues=upwash_clean(:,1)  Table=upwash_clean(:,9)
  enf_af : Lookup  InputValues=upwash_clean(:,1)  Table=upwash_clean(:,8)
  r2d : Fcn  Expr=u(1)*180/pi
  Out1 : Outport
  Out2 : Outport  Port=2
  wires:
  In4/1 -> r2d/1
  In3/1 -> [CL]
  In2/1 -> [Mach]
  d2r/1 -> Out1/1
  In1/1 -> Add/1
  average/1 -> d2r/1
  Get_eo/1 -> Mux/2
  Get_ei/1 -> Mux/1
  Mux/1 -> average/1
  Get_efo/1 -> Get_eo/2
  Get_en/1 -> Get_eo/3, Get_ei/3
  Get_efi/1 -> Get_ei/2
  en_an/1 -> Get_en/2
  Get_an/1 -> Get_en/1
  efo_af/1 -> Get_efo/1
  efi_af/1 -> Get_efi/1
  r2d/1 -> [alpha]
  [alpha] -> Get_an/3
  Get_enf/1 -> Get_an/1
  enf_af/1 -> Get_enf/2
  Get_af/1 -> Get_efo/2, Get_enf/1, Get_efi/2
  [Mach] -> enf_af/1
  [alpha] -> Get_af/2
  [CL] -> Get_enw/3(In2)
  [Mach] -> en_an/1, Get_enw/2(In3)
  [flap] -> Get_enw/1(In1)
  Get_enw/1(Out1) -> Get_an/2
  [CL] -> Get_efw/3(In2)
  [Mach] -> Get_efw/2(In3)
  [flap] -> Get_efw/1(In1)
  Get_efw/1(Out1) -> Get_af/1
  [Mach] -> efo_af/1, Get_ewo_CL/2(In3)
  [flap] -> Get_ewo_CL/1(In1)
  [Mach] -> efi_af/1, Get_ewi_CL/2(In3)
  [flap] -> Get_ewi_CL/1(In1)
  Constant/1 -> Add/2
  Add/1 -> [flap]
  Get_ewi/1 -> Get_ei/1
  Get_ewi_CL/1(Out1) -> Get_ewi/1, Mux1/1
  [CL] -> Get_ewi/2
  Get_ewo_CL/1(Out1) -> Get_ewo/1, Mux1/2
  Get_ewo/1 -> Get_eo/1
  [CL] -> Get_ewo/2
  Mux1/1 -> average1/1
  average1/1 -> d2r1/1
  d2r1/1 -> Out2/1

== system AssembledTEST1/Subsystem/Powerplants and Slipstream/Subsystem2/Powerplant - starboard (forces and moments about spinner) (in body axes)/Propeller - right (forces and moments about spinner) (in body axes)/Get air data at spinner ==
  In1 : Inport
  In2 : Inport  Port=2
  In3 : Inport  Port=3
  In4 : Inport  Port=4
  In5 : Inport  Port=5
  In6 : Inport  Port=6
  In7 : Inport  Port=7
  Add : Sum
  Display : Display
  Gain : Gain  Gain=-1
  Gain1 : Gain  Gain=-1
  Gain2 : Gain  Gain=-1
  Ground : Ground
  Ground1 : Ground
  Ground2 : Ground
  Matrix Concatenation{,1..3} (4 alike) : Concatenate  NumInputs=3  Mode=Multidimensional array
  Matrix Concatenation4 : Concatenate  NumInputs=3  Mode=Multidimensional array  ConcatenateDimension=2
  Mux2 : Mux  Inputs=2
  Product : Product  Inputs=**  Multiplication=Matrix(*)  RndMeth=Zero
  Trigonometric Function : Trigonometry
  Trigonometric Function1 : Trigonometry  Operator=cos
  Trigonometric Function2 : Trigonometry
  Trigonometric Function3 : Trigonometry  Operator=cos
  V_p : Fcn  Expr=sqrt(u(1)^2+u(2)^2+u(3)^2)
  alpha_p : Fcn  Expr=atan(u(4)/u(2))
  beta_p : Fcn  Expr=asin(u(3)/u(1))
  ub : Product  Inputs=3  RndMeth=Zero
  vb : Product  RndMeth=Zero
  wb : Product  Inputs=3  RndMeth=Zero
  Out1 : Outport
  Out3 : Outport  Port=2
  Out2 : Outport  Port=3
  wires:
  In2/1 -> Trigonometric Function1/1, Trigonometric Function/1
  In3/1 -> Trigonometric Function3/1, Trigonometric Function2/1
  Trigonometric Function1/1 -> ub/1
  Trigonometric Function3/1 -> ub/2, wb/2
  [V] -> ub/3
  Trigonometric Function/1 -> wb/1
  [V] -> wb/3
  Trigonometric Function2/1 -> vb/1
  [V] -> vb/2
  ub/1 -> Matrix Concatenation/1
  vb/1 -> Matrix Concatenation/2
  wb/1 -> Matrix Concatenation/3
  Ground/1 -> Matrix Concatenation1/1
  Gain/1 -> Matrix Concatenation1/3
  [r] -> Matrix Concatenation1/2
  [q] -> Gain/1
  [r] -> Gain1/1
  Gain1/1 -> Matrix Concatenation2/1
  Ground1/1 -> Matrix Concatenation2/2
  [p] -> Matrix Concatenation2/3
  [p] -> Gain2/1
  [q] -> Matrix Concatenation3/1
  Gain2/1 -> Matrix Concatenation3/2
  Ground2/1 -> Matrix Concatenation3/3
  Matrix Concatenation1/1 -> Matrix Concatenation4/1
  Matrix Concatenation2/1 -> Matrix Concatenation4/2
  Matrix Concatenation3/1 -> Matrix Concatenation4/3
  Matrix Concatenation4/1 -> Product/1
  Product/1 -> Add/2
  Matrix Concatenation/1 -> Add/1
  Add/1 -> V_p/1, Mux2/2
  V_p/1 -> Mux2/1, Out1/1
  Mux2/1 -> alpha_p/1, beta_p/1, Display/1
  In1/1 -> [V]
  In4/1 -> [p]
  In5/1 -> [q]
  alpha_p/1 -> Out2/1
  In6/1 -> [r]
  beta_p/1 -> Out3/1
  In7/1 -> Product/2

== system AssembledTEST1/Subsystem/Powerplants and Slipstream/Subsystem2/Powerplant - starboard (forces and moments about spinner) (in body axes)/Propeller - right (forces and moments about spinner) (in body axes)/propulsive//shaft ==
  In1 : Inport
  D0/q nacelles : Lookup  InputValues=pdrag_data(:,1)  Table=pdrag_data(:,6)
  Divide : Product  Inputs=*//
  Mux : Mux  Inputs=3
  alpha1 : Constant  Value=Ap
  alpha14 : Constant  Value=Sn
  alpha15 : Constant  Value=2
  propulsive/shaft : Fcn  Expr=1-(0.5*(u(3)/u(2))*((2.4*u(1))+0.51))
  Out1 : Outport
  wires:
  D0/q nacelles/1 -> Divide/1
  In1/1 -> D0/q nacelles/1
  alpha15/1 -> Divide/2
  alpha14/1 -> Divide/3, Mux/3
  Divide/1 -> Mux/1
  Mux/1 -> propulsive/shaft/1
  propulsive/shaft/1 -> Out1/1
  alpha1/1 -> Mux/2

== system AssembledTEST1/Subsystem/Powerplants and Slipstream/Subsystem2/Powerplant - starboard (forces and moments about spinner) (in body axes)/Propeller - right (forces and moments about spinner) (in body axes)/upwash at spinner ==
  In4 : Inport
  In1 : Inport  Port=2
  In3 : Inport  Port=3
  In2 : Inport  Port=4
  Add : Sum
  Constant : Constant
  Get_af : Sum
  Get_an : Sum  Inputs=+++
  Get_efi : Product  RndMeth=Zero
  Get_efo : Product  RndMeth=Zero
  Get_efw : Subsystem
      mask Display:
      | port_label('output',1,'\epsilon^f_{w}','texmode','on')
      | port_label('input',1,'flap')
      | port_label('input',2,'Mach')
      | port_label('input',3,'C_L','texmode','on')
  Get_ei : Sum  Inputs=+++
  Get_en : Product  RndMeth=Zero
  Get_enf : Product  RndMeth=Zero
  Get_enw : Subsystem
      mask Display:
      | port_label('output',1,'\epsilon^n_{w}','texmode','on')
      | port_label('input',1,'flap')
      | port_label('input',2,'Mach')
      | port_label('input',3,'C_L','texmode','on')
  Get_eo : Sum  Inputs=+++
  Get_ewi : Product  RndMeth=Zero
  Get_ewi_CL : Subsystem
      mask Display:
      | port_label('output',1,'\epsilon_{wi}/C_L','texmode','on')
      | port_label('input',1,'flap')
      | port_label('input',2,'Mach')
  Get_ewo : Product  RndMeth=Zero
  Get_ewo_CL : Subsystem
      mask Display:
      | port_label('output',1,'\epsilon_{wo}/C_L','texmode','on')
      | port_label('input',1,'flap')
      | port_label('input',2,'Mach')
  Mux : Mux  Inputs=2
  Mux1 : Mux  Inputs=2
  average : Fcn  Expr=0.5*(u(1)+u(2))
  average1 : Fcn  Expr=0.5*(u(1)+u(2))
  d2r : Fcn  Expr=u(1)*pi/180
  d2r1 : Fcn  Expr=u(1)*pi/180
  efi_af : Lookup  InputValues=upwash_clean(:,1)  Table=upwash_clean(:,6)
  efo_af : Lookup  InputValues=upwash_clean(:,1)  Table=upwash_clean(:,7)
  en_an : Lookup  InputValues=upwash_clean(:,1)  Table=upwash_clean(:,9)
  enf_af : Lookup  InputValues=upwash_clean(:,1)  Table=upwash_clean(:,8)
  r2d : Fcn  Expr=u(1)*180/pi
  Out1 : Outport
  Out2 : Outport  Port=2
  wires:
  In4/1 -> r2d/1
  In3/1 -> [CL]
  In2/1 -> [Mach]
  d2r/1 -> Out1/1
  In1/1 -> Add/1
  average/1 -> d2r/1
  Get_eo/1 -> Mux/2
  Get_ei/1 -> Mux/1
  Mux/1 -> average/1
  Get_efo/1 -> Get_eo/2
  Get_en/1 -> Get_eo/3, Get_ei/3
  Get_efi/1 -> Get_ei/2
  en_an/1 -> Get_en/2
  Get_an/1 -> Get_en/1
  efo_af/1 -> Get_efo/1
  efi_af/1 -> Get_efi/1
  r2d/1 -> [alpha]
  [alpha] -> Get_an/3
  Get_enf/1 -> Get_an/1
  enf_af/1 -> Get_enf/2
  Get_af/1 -> Get_efo/2, Get_enf/1, Get_efi/2
  [Mach] -> enf_af/1
  [alpha] -> Get_af/2
  [CL] -> Get_enw/3(In2)
  [Mach] -> en_an/1, Get_enw/2(In3)
  [flap] -> Get_enw/1(In1)
  Get_enw/1(Out1) -> Get_an/2
  [CL] -> Get_efw/3(In2)
  [Mach] -> Get_efw/2(In3)
  [flap] -> Get_efw/1(In1)
  Get_efw/1(Out1) -> Get_af/1
  [Mach] -> efo_af/1, Get_ewo_CL/2(In3)
  [flap] -> Get_ewo_CL/1(In1)
  [Mach] -> efi_af/1, Get_ewi_CL/2(In3)
  [flap] -> Get_ewi_CL/1(In1)
  Constant/1 -> Add/2
  Add/1 -> [flap]
  Get_ewi/1 -> Get_ei/1
  Get_ewi_CL/1(Out1) -> Get_ewi/1, Mux1/1
  [CL] -> Get_ewi/2
  Get_ewo_CL/1(Out1) -> Get_ewo/1, Mux1/2
  Get_ewo/1 -> Get_eo/1
  [CL] -> Get_ewo/2
  Mux1/1 -> average1/1
  average1/1 -> d2r1/1
  d2r1/1 -> Out2/1

== system AssembledTEST1/Subsystem/Powerplants and Slipstream/Subsystem2/Powerplant - port (forces and moments about spinner) (in body axes)/Propeller - left (forces and moments about spinner) (in body axes)/upwash at spinner/Get_efw ==
  In1 : Inport
  In3 : Inport  Port=2
  In2 : Inport  Port=3
  Multiport Switch : MultiPortSwitch  Inputs=4
  Product : Product  RndMeth=Zero
  efw_CL_clean : Lookup  InputValues=upwash_clean(:,1)  Table=upwash_clean(:,4)
  efw_CL_flaps10 : Lookup  InputValues=upwash_flaps(:,1)  Table=upwash_flaps(:,8)
  efw_CL_flaps20 : Lookup  InputValues=upwash_flaps(:,1)  Table=upwash_flaps(:,9)
  efw_CL_flaps35 : Lookup  InputValues=upwash_flaps(:,1)  Table=upwash_flaps(:,10)
  Out1 : Outport
  wires:
  In2/1 -> Product/2
  Product/1 -> Out1/1
  In1/1 -> Multiport Switch/1
  Multiport Switch/1 -> Product/1
  In3/1 -> efw_CL_clean/1, efw_CL_flaps10/1, efw_CL_flaps20/1, efw_CL_flaps35/1
  efw_CL_clean/1 -> Multiport Switch/2
  efw_CL_flaps10/1 -> Multiport Switch/3
  efw_CL_flaps20/1 -> Multiport Switch/4
  efw_CL_flaps35/1 -> Multiport Switch/5

== system AssembledTEST1/Subsystem/Powerplants and Slipstream/Subsystem2/Powerplant - port (forces and moments about spinner) (in body axes)/Propeller - left (forces and moments about spinner) (in body axes)/upwash at spinner/Get_enw ==
  In1 : Inport
  In3 : Inport  Port=2
  In2 : Inport  Port=3
  Multiport Switch : MultiPortSwitch  Inputs=4
  Product : Product  RndMeth=Zero
  enw_CL_clean : Lookup  InputValues=upwash_clean(:,1)  Table=upwash_clean(:,5)
  enw_CL_flaps10 : Lookup  InputValues=upwash_flaps(:,1)  Table=upwash_flaps(:,11)
  enw_CL_flaps20 : Lookup  InputValues=upwash_flaps(:,1)  Table=upwash_flaps(:,12)
  enw_CL_flaps35 : Lookup  InputValues=upwash_flaps(:,1)  Table=upwash_flaps(:,13)
  Out1 : Outport
  wires:
  In2/1 -> Product/2
  Product/1 -> Out1/1
  In1/1 -> Multiport Switch/1
  Multiport Switch/1 -> Product/1
  In3/1 -> enw_CL_clean/1, enw_CL_flaps10/1, enw_CL_flaps20/1, enw_CL_flaps35/1
  enw_CL_clean/1 -> Multiport Switch/2
  enw_CL_flaps10/1 -> Multiport Switch/3
  enw_CL_flaps20/1 -> Multiport Switch/4
  enw_CL_flaps35/1 -> Multiport Switch/5

== system AssembledTEST1/Subsystem/Powerplants and Slipstream/Subsystem2/Powerplant - port (forces and moments about spinner) (in body axes)/Propeller - left (forces and moments about spinner) (in body axes)/upwash at spinner/Get_ewi_CL ==
  In1 : Inport
  In3 : Inport  Port=2
  Multiport Switch : MultiPortSwitch  Inputs=4
  ewi_CL_clean : Lookup  InputValues=upwash_clean(:,1)  Table=upwash_clean(:,2)
  ewi_CL_flaps10 : Lookup  InputValues=upwash_flaps(:,1)  Table=upwash_flaps(:,2)
  ewi_CL_flaps20 : Lookup  InputValues=upwash_flaps(:,1)  Table=upwash_flaps(:,4)
  ewi_CL_flaps35 : Lookup  InputValues=upwash_flaps(:,1)  Table=upwash_flaps(:,6)
  Out1 : Outport
  wires:
  In1/1 -> Multiport Switch/1
  In3/1 -> ewi_CL_clean/1, ewi_CL_flaps10/1, ewi_CL_flaps20/1, ewi_CL_flaps35/1
  ewi_CL_clean/1 -> Multiport Switch/2
  ewi_CL_flaps10/1 -> Multiport Switch/3
  ewi_CL_flaps20/1 -> Multiport Switch/4
  ewi_CL_flaps35/1 -> Multiport Switch/5
  Multiport Switch/1 -> Out1/1

== system AssembledTEST1/Subsystem/Powerplants and Slipstream/Subsystem2/Powerplant - port (forces and moments about spinner) (in body axes)/Propeller - left (forces and moments about spinner) (in body axes)/upwash at spinner/Get_ewo_CL ==
  In1 : Inport
  In3 : Inport  Port=2
  Multiport Switch : MultiPortSwitch  Inputs=4
  ewo_CL_clean : Lookup  InputValues=upwash_clean(:,1)  Table=upwash_clean(:,3)
  ewo_CL_flaps10 : Lookup  InputValues=upwash_flaps(:,1)  Table=upwash_flaps(:,3)
  ewo_CL_flaps20 : Lookup  InputValues=upwash_flaps(:,1)  Table=upwash_flaps(:,5)
  ewo_CL_flaps35 : Lookup  InputValues=upwash_flaps(:,1)  Table=upwash_flaps(:,7)
  Out1 : Outport
  wires:
  In1/1 -> Multiport Switch/1
  In3/1 -> ewo_CL_clean/1, ewo_CL_flaps10/1, ewo_CL_flaps20/1, ewo_CL_flaps35/1
  ewo_CL_clean/1 -> Multiport Switch/2
  ewo_CL_flaps10/1 -> Multiport Switch/3
  ewo_CL_flaps20/1 -> Multiport Switch/4
  ewo_CL_flaps35/1 -> Multiport Switch/5
  Multiport Switch/1 -> Out1/1

== system AssembledTEST1/Subsystem/Powerplants and Slipstream/Subsystem2/Powerplant - starboard (forces and moments about spinner) (in body axes)/Propeller - right (forces and moments about spinner) (in body axes)/upwash at spinner/Get_efw ==
  In1 : Inport
  In3 : Inport  Port=2
  In2 : Inport  Port=3
  Multiport Switch : MultiPortSwitch  Inputs=4
  Product : Product  RndMeth=Zero
  efw_CL_clean : Lookup  InputValues=upwash_clean(:,1)  Table=upwash_clean(:,4)
  efw_CL_flaps10 : Lookup  InputValues=upwash_flaps(:,1)  Table=upwash_flaps(:,8)
  efw_CL_flaps20 : Lookup  InputValues=upwash_flaps(:,1)  Table=upwash_flaps(:,9)
  efw_CL_flaps35 : Lookup  InputValues=upwash_flaps(:,1)  Table=upwash_flaps(:,10)
  Out1 : Outport
  wires:
  In2/1 -> Product/2
  Product/1 -> Out1/1
  In1/1 -> Multiport Switch/1
  Multiport Switch/1 -> Product/1
  In3/1 -> efw_CL_clean/1, efw_CL_flaps10/1, efw_CL_flaps20/1, efw_CL_flaps35/1
  efw_CL_clean/1 -> Multiport Switch/2
  efw_CL_flaps10/1 -> Multiport Switch/3
  efw_CL_flaps20/1 -> Multiport Switch/4
  efw_CL_flaps35/1 -> Multiport Switch/5

== system AssembledTEST1/Subsystem/Powerplants and Slipstream/Subsystem2/Powerplant - starboard (forces and moments about spinner) (in body axes)/Propeller - right (forces and moments about spinner) (in body axes)/upwash at spinner/Get_enw ==
  In1 : Inport
  In3 : Inport  Port=2
  In2 : Inport  Port=3
  Multiport Switch : MultiPortSwitch  Inputs=4
  Product : Product  RndMeth=Zero
  enw_CL_clean : Lookup  InputValues=upwash_clean(:,1)  Table=upwash_clean(:,5)
  enw_CL_flaps10 : Lookup  InputValues=upwash_flaps(:,1)  Table=upwash_flaps(:,11)
  enw_CL_flaps20 : Lookup  InputValues=upwash_flaps(:,1)  Table=upwash_flaps(:,12)
  enw_CL_flaps35 : Lookup  InputValues=upwash_flaps(:,1)  Table=upwash_flaps(:,13)
  Out1 : Outport
  wires:
  In2/1 -> Product/2
  Product/1 -> Out1/1
  In1/1 -> Multiport Switch/1
  Multiport Switch/1 -> Product/1
  In3/1 -> enw_CL_clean/1, enw_CL_flaps10/1, enw_CL_flaps20/1, enw_CL_flaps35/1
  enw_CL_clean/1 -> Multiport Switch/2
  enw_CL_flaps10/1 -> Multiport Switch/3
  enw_CL_flaps20/1 -> Multiport Switch/4
  enw_CL_flaps35/1 -> Multiport Switch/5

== system AssembledTEST1/Subsystem/Powerplants and Slipstream/Subsystem2/Powerplant - starboard (forces and moments about spinner) (in body axes)/Propeller - right (forces and moments about spinner) (in body axes)/upwash at spinner/Get_ewi_CL ==
  In1 : Inport
  In3 : Inport  Port=2
  Multiport Switch : MultiPortSwitch  Inputs=4
  ewi_CL_clean : Lookup  InputValues=upwash_clean(:,1)  Table=upwash_clean(:,2)
  ewi_CL_flaps10 : Lookup  InputValues=upwash_flaps(:,1)  Table=upwash_flaps(:,2)
  ewi_CL_flaps20 : Lookup  InputValues=upwash_flaps(:,1)  Table=upwash_flaps(:,4)
  ewi_CL_flaps35 : Lookup  InputValues=upwash_flaps(:,1)  Table=upwash_flaps(:,6)
  Out1 : Outport
  wires:
  In1/1 -> Multiport Switch/1
  In3/1 -> ewi_CL_clean/1, ewi_CL_flaps10/1, ewi_CL_flaps20/1, ewi_CL_flaps35/1
  ewi_CL_clean/1 -> Multiport Switch/2
  ewi_CL_flaps10/1 -> Multiport Switch/3
  ewi_CL_flaps20/1 -> Multiport Switch/4
  ewi_CL_flaps35/1 -> Multiport Switch/5
  Multiport Switch/1 -> Out1/1

== system AssembledTEST1/Subsystem/Powerplants and Slipstream/Subsystem2/Powerplant - starboard (forces and moments about spinner) (in body axes)/Propeller - right (forces and moments about spinner) (in body axes)/upwash at spinner/Get_ewo_CL ==
  In1 : Inport
  In3 : Inport  Port=2
  Multiport Switch : MultiPortSwitch  Inputs=4
  ewo_CL_clean : Lookup  InputValues=upwash_clean(:,1)  Table=upwash_clean(:,3)
  ewo_CL_flaps10 : Lookup  InputValues=upwash_flaps(:,1)  Table=upwash_flaps(:,3)
  ewo_CL_flaps20 : Lookup  InputValues=upwash_flaps(:,1)  Table=upwash_flaps(:,5)
  ewo_CL_flaps35 : Lookup  InputValues=upwash_flaps(:,1)  Table=upwash_flaps(:,7)
  Out1 : Outport
  wires:
  In1/1 -> Multiport Switch/1
  In3/1 -> ewo_CL_clean/1, ewo_CL_flaps10/1, ewo_CL_flaps20/1, ewo_CL_flaps35/1
  ewo_CL_clean/1 -> Multiport Switch/2
  ewo_CL_flaps10/1 -> Multiport Switch/3
  ewo_CL_flaps20/1 -> Multiport Switch/4
  ewo_CL_flaps35/1 -> Multiport Switch/5
  Multiport Switch/1 -> Out1/1

== matlab function AssembledTEST1/Equations of Motion/Navigation_equations/DCM_matrix ==
  data: EUL input; T output
function T  = DCM(EUL)

%Euler Angles
Phi   = EUL(1);
Theta = EUL(2);
Psi   = EUL(3);

%% Cosine Matrix

T = zeros (3,3);

T(1,1) = cos(Theta)*cos(Psi);
T(1,2) = cos(Theta)*sin(Psi);
T(1,3) = -sin(Theta);

T(2,1) = -cos(Phi)*sin(Psi) + sin(Phi)*sin(Theta)*cos(Psi);
T(2,2) = cos(Phi)*cos(Psi) +sin(Phi)*sin(Theta)*sin(Psi);
T(2,3) = sin(Phi)*cos(Theta);

T(3,1) = sin(Phi)*sin(Psi) + cos(Phi)*sin(Theta)*cos(Psi);
T(3,2) = -sin(Phi)*cos(Psi)+ cos(Phi)*sin(Theta)*sin(Psi);
T(3,3) = cos(Phi)*cos(Theta);
end

== matlab function AssembledTEST1/Equations of Motion/EoMs ==
  data: Forces input; Vdot output; Moments input; velocity input; omega input; omegadot output; MASS input; INERTIA input; CG input
function [Vdot,omegadot]= Equations_of_Motion(Forces,Moments,velocity,omega,MASS,INERTIA,CG)
%Variable definition
m=MASS;
dx=CG(1);
dy=CG(2);
dz=CG(3);
I=INERTIA;
Ixx=I(1,1);
Iyy=I(2,2);
Izz=I(3,3);
Ixz=I(1,3);


U=velocity(1);
V=velocity(2);
W=velocity(3);

P=omega(1);
Q=omega(2);
R=omega(3);


X=Forces(1);
Y=Forces(2);
Z=Forces(3);

L=Moments(1);
M=Moments(2);
N=Moments(3);

% Motion's Matrix composition


massProperties=[
        m       0       0       0       m*dz   -m*dy;
        0       m       0      -m*dz    0       m*dx;
        0       0       m       m*dy   -m*dx    0   ;
        0      -m*dz    m*dy    Ixx     0      -Ixz ;
        m*dz    0      -m*dx    0       Iyy     0   ;
       -m*dy    m*dx    0      -Ixz     0       Izz  ];
   
dynamicProperties=[
        X+m*R*V-m*Q*W+m*dx*(Q^2+R^2)-m*dy*P*Q-m*dz*P*R;
        Y-m*R*U+m*P*W-m*dx*P*Q+m*dy*(P^2+R^2)-m*dz*Q*R;
        Z+m*Q*U-m*P*V-m*dx*P*R+m*dy*Q*R+m*dz*(P^2+Q^2);
        L-Q*R*(Izz-Iyy)+P*Q*Ixz-(P*V-Q*U)*m*dy+(R*U-P*W)*m*dz;
        M-P*R*(Ixx-Izz)-(P^2-R^2)*Ixz-(Q*U-P*V)*m*dx-(Q*W-R*V)*m*dz;
        N-P*Q*(Iyy-Ixx)-Q*R*Ixz-(R*U-P*W)*m*dx+(Q*W-R*V)*m*dy];
 
% Motion output
    
motion=massProperties\dynamicProperties;  


Vdot        =motion(1:3);
omegadot    =motion(4:6);

%Problemes:
%dx in angular

end
